simulink model "Gyro_Heading_Estimation"  (R2019a)
settings: Solver=ode3  StartTime=0.0  StopTime=inf  FixedStep=0.002  RelTol=1e-3  EnableMultiTasking=on
undefined symbols (not defined in the file): HIL, qc_get_step_size
libraries: quarc_library x12, simulink x8
settings Model: SimulationMode=external  ExtModeTrigDuration=10000  Creator=Derek  LastModifiedBy=Derek
settings SolverCC: PositivePriorityOrder=on
settings DataIOCC: ReturnWorkspaceOutputs=off
settings DebuggingCC: ArithmeticOperatorsInVariantConditions=warning
settings HardwareCC: ProdBitPerLong=64  ProdLargestAtomicInteger=LongLong  ProdLargestAtomicFloat=Double  ProdLongLongMode=on  ProdHWDeviceType=ARM Compatible->ARM 64-bit (LP64)
settings SFSimCC: SimUseLocalCustomCode=off
settings RTWCC: SystemTargetFile=quarc_linux_nvidia.tlc  TemplateMakefile=quarc_default_tmf  Description=QUARC Linux Nvidia Target (QCar) Using Toolchain  RTWUseLocalCustomCode=off  Toolchain=QUARC linux_nvidia | gmake (64-bit Windows)  BuildConfiguration=Faster Runs
settings CodeAppCC: StateflowObjectComments=on
settings STFCustomTargetCC: TargetLangStandard=C99 (ISO)  ConcurrentExecutionCompliant=on  UseToolchainInfoCompliant=on  SystemTargetFile=quarc_linux_nvidia.tlc
settings GRTTargetCC: ParMdlRefBuildCompliant=off  CompOptLevelCompliant=off  CombineOutputUpdateFcns=off  MatFileLogging=off  CPPClassGenCompliant=off  GRTInterface=on  ExtMode=on  ExtModeMexFile=quarc_comm  ExtModeMexArgs='-w -d /tmp -uri %u'
settings ConfigComp: CovMetricSettings=dswe

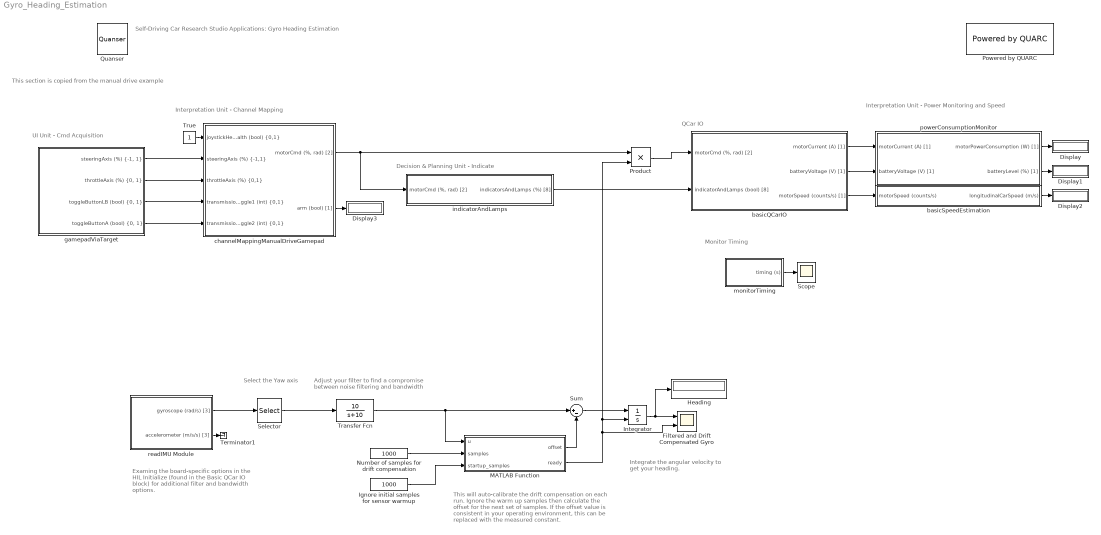
== system Gyro_Heading_Estimation ==
  note: Select the Yaw axis
  note: Decision & Planning Unit - Indicate
  note: Interpretation Unit - Power Monitoring and Speed
  note: QCar IO
  note: UI Unit - Cmd Acquisition
  note: Monitor Timing
  note: Interpretation Unit - Channel Mapping
  note: Self-Driving Car Research Studio
      | Applications: Gyro Heading Estimation
  note: This section is copied from the manual drive example
  note: Adjust your filter to find a compromise
      | between noise filtering and bandwidth
  note: This will auto-calibrate the drift compensation
      | on each run. Ignore the warm up samples
      | then calculate the offset for the next set of samples.
      | If the offset value is consistent in your operating
      | environment, this can be replaced with the measured
      | constant.
  note: Integrate the angular velocity to
      | get your heading.
  note: Examing the board-specific options
      | in the HIL Initialize (found in the Basic
      | QCar IO block) for additional filter
      | and bandwidth options.
  Display{,1..3} (4 alike) : Display
      Display settings: Decimation=0.5/qc_get_step_size
      Display1 settings: Decimation=0.5/qc_get_step_size
      Display2 settings: Decimation=0.5/qc_get_step_size
      Display3 settings: Decimation=0.1/qc_get_step_size
  Filtered and Drift Compensated Gyro : Scope  NumInputPorts=2
  Heading : Display
  Ignore initial samples for sensor warmup : Constant  Value=1000
  Integrator : Integrator  ExternalReset=rising
  MATLAB Function : MATLAB Function  TreatAsAtomicUnit=on
  Number of samples for drift compensation : Constant  Value=1000
  Powered by QUARC : quarc_library/Logos/Powered by QUARC
  Product : Product
  Quanser : quarc_library/Logos/Quanser
  Scope : Scope
  Selector : Selector  InputPortWidth=3  IndexOptions=Index vector (dialog)  Indices=[3]  OutputSizes=1
  Sum : Sum  Inputs=|+-
  Terminator1 : Terminator
  Transfer Fcn : TransferFcn  Numerator=[10]  Denominator=[1 10]
  True : Constant
  basicQCarIO : Subsystem
  basicSpeedEstimation : Subsystem
  channelMappingManualDriveGamepad : Subsystem
  gamepadViaTarget : Subsystem
  indicatorAndLamps : Subsystem
  "monitorTiming " : Subsystem
  powerConsumptionMonitor : Subsystem
  readIMU Module : Subsystem
  wires:
  readIMU Module/1(gyroscope (rad/s) [3]) -> Selector/1
  readIMU Module/2(accelerometer (m/s/s) [3]) -> Terminator1/1
  Selector/1 -> Transfer Fcn/1
  Transfer Fcn/1 -> Sum/1, MATLAB Function/1(u)
  Integrator/1 -> Heading/1, Filtered and Drift Compensated Gyro/1
  Sum/1 -> Integrator/1
  MATLAB Function/1(offset) -> Sum/2
  MATLAB Function/2(ready) -> Filtered and Drift Compensated Gyro/2, Product/2, Integrator/2
  Number of samples for drift compensation/1 -> MATLAB Function/2(samples)
  Ignore initial samples for sensor warmup/1 -> MATLAB Function/3(startup_samples)
  basicQCarIO/3(motorSpeed (counts/s) [1]) -> basicSpeedEstimation/1(motorSpeed (counts/s))
  gamepadViaTarget/4("toggleButtonA (bool) {0, 1}") -> channelMappingManualDriveGamepad/5("transmissionToggle2 (int) {0,1}")
  True/1 -> channelMappingManualDriveGamepad/1("joystickHealth (bool) {0,1}")
  gamepadViaTarget/1("steeringAxis (%) {-1, 1}") -> channelMappingManualDriveGamepad/2("steeringAxis (%) {-1,1}")
  basicQCarIO/1(motorCurrent (A) [1]) -> powerConsumptionMonitor/1(motorCurrent (A) [1])
  gamepadViaTarget/3("toggleButtonLB (bool) {0, 1}") -> channelMappingManualDriveGamepad/4("transmissionToggle1 (int) {0,1}")
  powerConsumptionMonitor/1(motorPowerConsumption (W) [1]) -> Display/1
  powerConsumptionMonitor/2(batteryLevel (%) [1]) -> Display1/1
  gamepadViaTarget/2("throttleAxis (%) {0, 1}") -> channelMappingManualDriveGamepad/3("throttleAxis (%) {0,1}")
  channelMappingManualDriveGamepad/1("motorCmd (%, rad) [2]") -> indicatorAndLamps/1("motorCmd (%, rad) [2]"), Product/1
  basicQCarIO/2(batteryVoltage (V) [1]) -> powerConsumptionMonitor/2(batteryVoltage (V) [1])
  basicSpeedEstimation/1(longitudinalCarSpeed (m/s)) -> Display2/1
  channelMappingManualDriveGamepad/2(arm (bool) [1]) -> Display3/1
  "monitorTiming "/1(timing (s)) -> Scope/1
  indicatorAndLamps/1(indicatorsAndLamps (%) [8]) -> basicQCarIO/2(indicatorAndLamps (bool) [8])
  Product/1 -> basicQCarIO/1("motorCmd (%, rad) [2]")

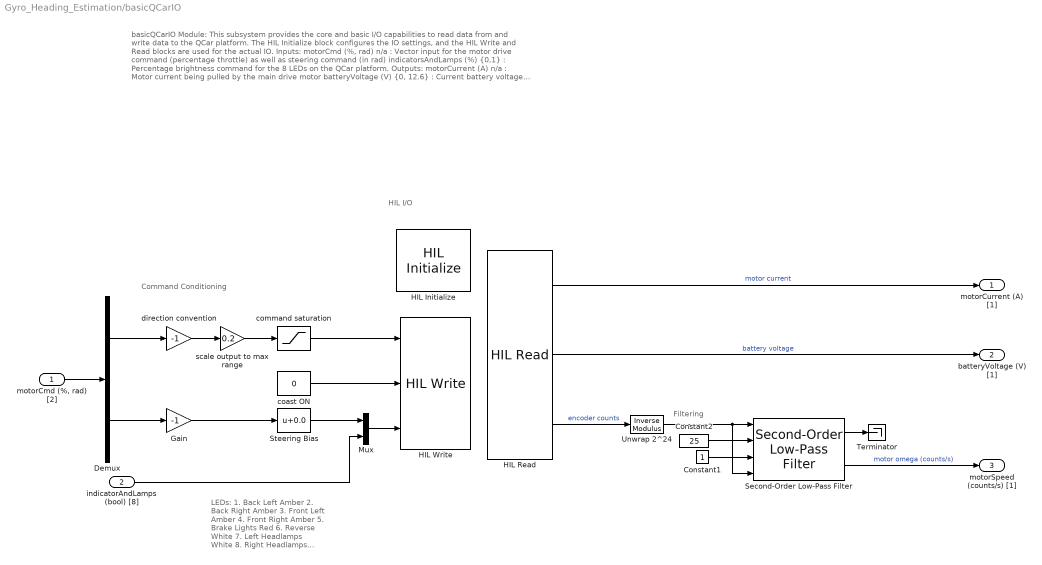
== system Gyro_Heading_Estimation/basicQCarIO ==
  note: Filtering
  note: basicQCarIO Module:
      |
      | This subsystem provides the core and basic I/O capabilities to read data from and write data to the QCar platform. The HIL Initialize block configures the IO settings, and the HIL Write and Read blocks are used for the actual IO.
      |
      | Inputs:
      | motorCmd (%, rad) n/a : Vector input for the motor drive command (percentage throttle) as well as steering command (in rad)
      | indicatorsAndLamps (%) {0,1} : Percentage brightness command for the 8 LEDs on the QCar platform.
      |
      | Outputs:
      | motorCurrent (A) n/a : Motor current being pulled by the main drive motor
      | batteryVoltage (V) {0, 12.6} : Current battery voltage reading
      | motorSpeed (counts/s) n/a : Drive motor speed measured using an encoder (do not confuse with wheel speed as this measurement is at the drive shaft)
  note: Command Conditioning
  note: HIL I/O
  note: LEDs:
      | 1. Back Left Amber
      | 2. Back Right Amber
      | 3. Front Left Amber
      | 4. Front Right Amber
      | 5. Brake Lights Red
      | 6. Reverse White
      | 7. Left Headlamps White
      | 8. Right Headlamps White
  "motorCmd (%, rad) [2]" : Inport
  indicatorAndLamps (bool) [8] : Inport  Port=2
  Constant1 : Constant
  Constant2 : Constant  Value=25
  Demux : Demux  Outputs=2
  Gain : Gain  Gain=-1
  HIL Initialize : quarc_library/Data Acquisition/Generic/Configuration/HIL Initialize  object_name=HIL-2  board_type=qcar  board_number=0  board_options=gyro_fs=250;gyro_rate=64;accel_fs=2;accel_rate=62.5;mag_rate=20;mag_xy=47;mag_z=83;enc1_dir=0;enc2_dir=0;enc3_dir=0;enc4_dir=0;pwm1_dshot=0;pwm2_dshot=0;pwm3_dshot=0;pwm4_dshot=0;pwm5_dshot=0;pwm6_dshot=0;pwm7_dshot=0;steer_bias=0.05;motor_limit=0.3;  exclusive=off  active=on  hardware_clocks=[]  clock_modes=[]  initial_clock_frequencies=[]  set_clock_params_at_start=off  set_clock_params_at_switch_in=off  set_clock_frequencies_at_start=off  set_clock_frequencies_at_switch_in=off  analog_input_channels=[0:6]  analog_input_configurations=[]  analog_input_maximums=[3.3]  analog_input_minimums=[0]  set_analog_input_params_at_start=off  set_analog_input_params_at_switch_in=off  analog_output_channels=[]  analog_output_maximums=[]  analog_output_minimums=[]  initial_analog_outputs=[]  final_analog_outputs=[]  watchdog_analog_outputs=[]  set_analog_output_params_at_start=off  set_analog_output_params_at_switch_in=off  set_analog_outputs_at_start=off  set_analog_outputs_at_switch_in=off  set_analog_outputs_at_terminate=off  set_analog_outputs_at_switch_out=off  set_analog_outputs_on_watchdog=off  digital_input_channels=[24:43]  digital_output_channels=[40]  digital_output_configuration=[]  initial_digital_outputs=[0]  final_digital_outputs=[1]  watchdog_digital_outputs=[]  set_digital_output_params_at_start=off  set_digital_output_params_at_switch_in=off  set_digital_outputs_at_start=on  set_digital_outputs_at_switch_in=off  set_digital_outputs_at_terminate=on  set_digital_outputs_at_switch_out=off  set_digital_outputs_on_watchdog=off  encoder_channels=[0:4]  quadrature=[4 4]  encoder_filter_frequency=100e6/1  initial_encoder_counts=[0]  set_encoder_params_at_start=on  set_encoder_params_at_switch_in=off  set_encoder_counts_at_start=on  set_encoder_counts_at_switch_in=off  pwm_channels=[0:7]  pwm_modes=[0 0]  pwm_frequency=150e6/4096  pwm_configuration=[0]  pwm_alignment=[0]  pwm_polarity=[1]  pwm_leading_deadband=[]  pwm_trailing_deadband=[]  initial_pwm_outputs=[0]  final_pwm_outputs=[0]  watchdog_pwm_outputs=[0]  set_pwm_params_at_start=on  set_pwm_params_at_switch_in=off  set_pwm_outputs_at_start=on  set_pwm_outputs_at_switch_in=off  set_pwm_outputs_at_terminate=on  set_pwm_outputs_at_switch_out=off  set_pwm_outputs_on_watchdog=off  other_output_channels=[1000, 11000:11011]  initial_other_outputs=[0]  final_other_outputs=[0]  watchdog_other_outputs=[]  set_other_outputs_at_start=on  set_other_outputs_at_switch_in=off  set_other_outputs_at_terminate=on  set_other_outputs_at_switch_out=off  set_other_outputs_on_watchdog=off
  HIL Read : quarc_library/Data Acquisition/Generic/Immediate I//O/HIL Read  object_name=HIL-2  analog_channels=[5:6]  encoder_channels=[0]  digital_channels=[]  other_channels=[]  sample_time=qc_get_step_size  active=on  vector_output=off  data_type_mode=Inherit via back propagation  encoder_data_type=double  digital_data_type=boolean
  HIL Write : quarc_library/Data Acquisition/Generic/Immediate I//O/HIL Write  object_name=HIL-2  analog_channels=[]  pwm_channels=[0]  digital_channels=[40]  other_channels=[1000 11008:11011 11000:11003]  sample_time=-1  active=off  vector_input=on
  Mux : Mux  Inputs=2
  Second-Order Low-Pass Filter : quarc_library/Continuous/Second-Order Low-Pass Filter  params_source=External (input ports)  input_width=1  input_zeta=1  input_init=0
  Steering Bias : Bias  Bias=0.0
  Terminator : Terminator
  Unwrap 2^24 : quarc_library/Discontinuities/Inverse Modulus  modulus=16777215  output_derivative=off  output_revolutions=off  max_x=Inf  min_x=-Inf
  coast ON : Constant  Value=0
  command saturation : Saturate  UpperLimit=0.20  LowerLimit=-0.20
  direction convention : Gain  Gain=-1
  scale output to max range : Gain  Gain=0.2
  motorCurrent (A) [1] : Outport
  batteryVoltage (V) [1] : Outport  Port=2
  motorSpeed (counts/s) [1] : Outport  Port=3
  wires:
  Constant2/1 -> Second-Order Low-Pass Filter/2
  Unwrap 2^24/1 -> Second-Order Low-Pass Filter/1, Second-Order Low-Pass Filter/4
  Demux/2 -> Gain/1
  direction convention/1 -> scale output to max range/1
  "motorCmd (%, rad) [2]"/1 -> Demux/1
  command saturation/1 -> HIL Write/1
  coast ON/1 -> HIL Write/2
  Second-Order Low-Pass Filter/1 -> Terminator/1
  indicatorAndLamps (bool) [8]/1 -> Mux/2
  Steering Bias/1 -> Mux/1
  Mux/1 -> HIL Write/3
  Second-Order Low-Pass Filter/2 -> motorSpeed (counts/s) [1]/1  "motor omega (counts/s)"
  Constant1/1 -> Second-Order Low-Pass Filter/3
  Demux/1 -> direction convention/1
  HIL Read/3 -> Unwrap 2^24/1  "encoder counts"
  Gain/1 -> Steering Bias/1
  HIL Read/1 -> motorCurrent (A) [1]/1  "motor current"
  HIL Read/2 -> batteryVoltage (V) [1]/1  "battery voltage"
  scale output to max range/1 -> command saturation/1

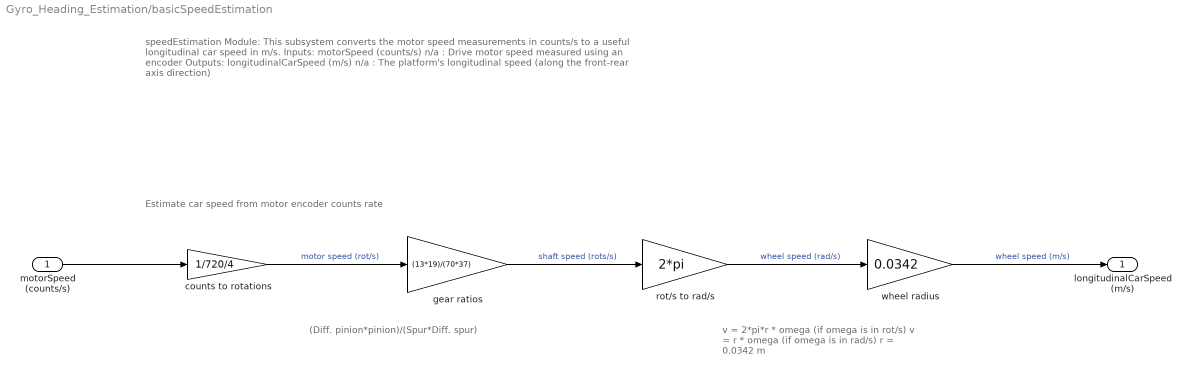
== system Gyro_Heading_Estimation/basicSpeedEstimation ==
  note: speedEstimation Module:
      |
      | This subsystem converts the motor speed measurements in counts/s to a useful longitudinal car speed in m/s.
      |
      | Inputs:
      | motorSpeed (counts/s) n/a : Drive motor speed measured using an encoder
      |
      | Outputs:
      | longitudinalCarSpeed (m/s) n/a : The platform's longitudinal speed (along the front-rear axis direction)
  note: (Diff. pinion*pinion)/(Spur*Diff. spur)
  note: v = 2*pi*r * omega (if omega is in rot/s)
      | v = r * omega (if omega is in rad/s)
      | r = 0.0342 m
  note: Estimate car speed from motor encoder counts rate
  motorSpeed (counts/s) : Inport
  counts to rotations : Gain  Gain=1/720/4
  gear ratios : Gain  Gain=(13*19)/(70*37)
  rot/s to rad/s : Gain  Gain=2*pi
  wheel radius : Gain  Gain=0.0342
  longitudinalCarSpeed (m/s) : Outport
  wires:
  gear ratios/1 -> rot/s to rad/s/1  "shaft speed (rots/s)"
  wheel radius/1 -> longitudinalCarSpeed (m/s)/1  "wheel speed (m/s)"
  counts to rotations/1 -> gear ratios/1  "motor speed (rot/s)"
  rot/s to rad/s/1 -> wheel radius/1  "wheel speed (rad/s)"
  motorSpeed (counts/s)/1 -> counts to rotations/1

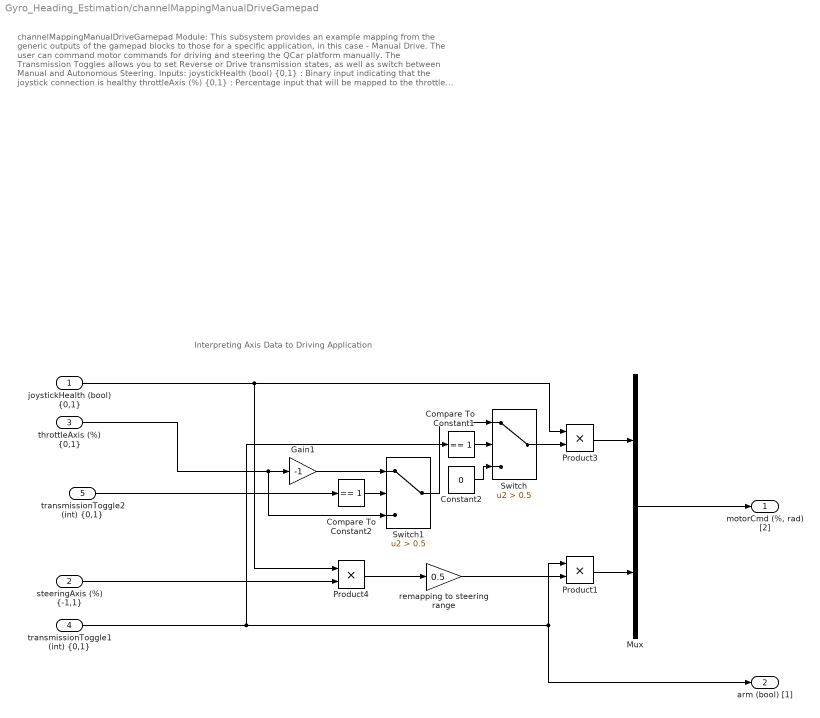
== system Gyro_Heading_Estimation/channelMappingManualDriveGamepad ==
  note: channelMappingManualDriveGamepad Module:
      |
      | This subsystem provides an example mapping from the generic outputs of the gamepad blocks to those for a specific application, in this case - Manual Drive. The user can command motor commands for driving and steering the QCar platform manually. The Transmission Toggles allows you to set Reverse or Drive transmission states, as well as switch between Manual and Autonomous Steering.
      |
      | Inputs:
      | joystickHealth (bool) {0,1} : Binary input indicating that the joystick connection is healthy
      | throttleAxis (%) {0,1} : Percentage input that will be mapped to the throttle command
      | steeringAxis (%) {-1,1} : Signed percentage input that will be mapped to steering
      | transmissionToggle1 (int) {0,1} : 2-state input that will decide the Park/Engage State
      | transmissionToggle2 (int) {0, 1} : 2-state input that will decide the Reverse/Drive State
      |
      | Outputs:
      | motorCmd (%, rad) n/a : Vector output for the motor drive command (percentage throttle) as well as steering command (in rad)
      | arm (bool) {0,1} : Binary output indicating status (armed or disarmed)
      |
      | Usage:
      | 1. When the Transmission Toggle 1 input
      | a. reads 1, the Arm output will be high (1), which is the Armed state.
      | b. reads 0, the Arm output will be low (0), which is the Disarmed state.
      | 2. In addition, the Transmission Toggle 2 input
      | a. reading 0 is the Drive state, and the Motor Cmd for the throttle will range from 0 to 100%, spinning the wheels forwards.
      | b. reading 1 is the Reverse state, and the Motor Cmd for the throttle will range from 0 to -100%, spinning the wheels backwards.
  note: Interpreting Axis Data to Driving Application
  "joystickHealth (bool) {0,1}" : Inport
  "steeringAxis (%) {-1,1}" : Inport  Port=2
  "throttleAxis (%) {0,1}" : Inport  Port=3
  "transmissionToggle1 (int) {0,1}" : Inport  Port=4
  "transmissionToggle2 (int) {0,1}" : Inport  Port=5
  " remapping to steering range " : Gain  Gain=0.5
  Compare To Constant1 : simulink/Logic and Bit Operations/Compare To Constant  relop===  const=1  OutDataTypeStr=boolean
  Compare To Constant2 : simulink/Logic and Bit Operations/Compare To Constant  relop===  const=1  OutDataTypeStr=boolean
  Constant2 : Constant  Value=0
  Gain1 : Gain  Gain=-1
  Mux : Mux  Inputs=2
  Product1 : Product
  Product3 : Product
  Product4 : Product
  Switch : Switch  Criteria=u2 > Threshold  Threshold=0.5
  Switch1 : Switch  Criteria=u2 > Threshold  Threshold=0.5
  "motorCmd (%, rad) [2]" : Outport
  arm (bool) [1] : Outport  Port=2
  wires:
  Switch/1 -> Product3/2
  Product1/1 -> Mux/2
  Compare To Constant1/1 -> Switch/2
  "steeringAxis (%) {-1,1}"/1 -> Product4/2
  "joystickHealth (bool) {0,1}"/1 -> Product4/1, Product3/1
  "transmissionToggle1 (int) {0,1}"/1 -> Compare To Constant1/1, Product1/1, arm (bool) [1]/1
  Product3/1 -> Mux/1
  " remapping to steering range "/1 -> Product1/2
  Product4/1 -> " remapping to steering range "/1
  "throttleAxis (%) {0,1}"/1 -> Switch1/3, Gain1/1
  Mux/1 -> "motorCmd (%, rad) [2]"/1
  Compare To Constant2/1 -> Switch1/2
  Switch1/1 -> Switch/1
  Constant2/1 -> Switch/3
  "transmissionToggle2 (int) {0,1}"/1 -> Compare To Constant2/1
  Gain1/1 -> Switch1/1

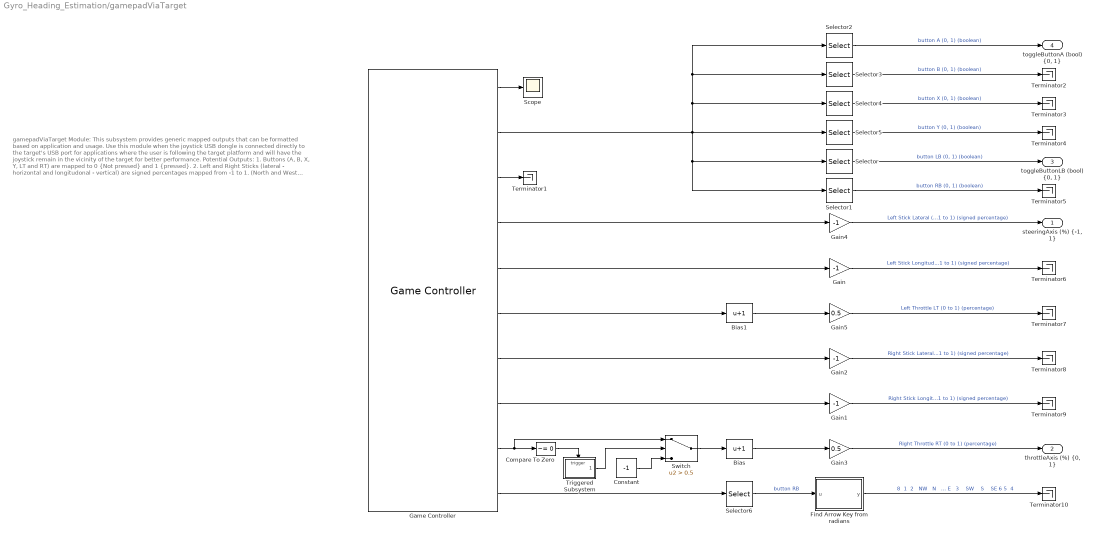
== system Gyro_Heading_Estimation/gamepadViaTarget ==
  note: gamepadViaTarget Module:
      |
      | This subsystem provides generic mapped outputs that can be formatted based on application and usage. Use this module when the joystick USB dongle is connected directly to the target's USB port for applications where the user is following the target platform and will have the joystick remain in the vicinity of the target for better performance.
      |
      | Potential Outputs:
      |
      | 1. Buttons (A, B, X, Y, LT and RT) are mapped to 0 {Not pressed} and 1 {pressed}.
      |
      | 2. Left and Right Sticks (lateral - horizontal and longitudonal - vertical) are signed percentages mapped from -1 to 1. (North and West directions are positive)
      |
      | 3. Throttle (RT and LT) are mapped from 0 to 1.
      |
      | 4. Arrow keys are mapped to constants 1 to 8 starting from North and incrementing clockwise up to North West. A value of 0 implies no keys are pressed.
      |
      | 5. The NEW signal triggers a high (1) pulse whenever a value on any of the gamepad's keys changes.
      |
      | NOTE: The Gamepad F710 dongle MUST be plugged into the target's USB port to use this module.
  Bias : Bias  Bias=1
  Bias1 : Bias  Bias=1
  Compare To Zero : simulink/Logic and Bit Operations/Compare To Zero  relop=~=  OutDataTypeStr=boolean
  Constant : Constant  Value=-1
  Find Arrow Key from radians : MATLAB Function  TreatAsAtomicUnit=on
  Gain{,1..2,4} (4 alike) : Gain  Gain=-1
  Gain3 : Gain  Gain=0.5
  Gain5 : Gain  Gain=0.5
  Game Controller : quarc_library/Devices/Peripherals/Target/Game Controller  controller=1  buffer_size=12  deadzone=[]  saturation=[]  sample_time=qc_get_step_size  auto_center=off  enabled=on
      settings: SourceProductName=QUARC Targets
  Scope : Scope
  Selector : Selector  InputPortWidth=32  IndexOptions=Index vector (dialog)  Indices=[5]  OutputSizes=1
  Selector1 : Selector  InputPortWidth=32  IndexOptions=Index vector (dialog)  Indices=[6]  OutputSizes=1
  Selector2 : Selector  InputPortWidth=32  IndexOptions=Index vector (dialog)  Indices=[1]  OutputSizes=1
  Selector3 : Selector  InputPortWidth=32  IndexOptions=Index vector (dialog)  Indices=[2]  OutputSizes=1
  Selector4 : Selector  InputPortWidth=32  IndexOptions=Index vector (dialog)  Indices=[3]  OutputSizes=1
  Selector5 : Selector  InputPortWidth=32  IndexOptions=Index vector (dialog)  Indices=[4]  OutputSizes=1
  Selector6 : Selector  InputPortWidth=4  IndexOptions=Index vector (dialog)  Indices=[1]  OutputSizes=1
  Switch : Switch  Criteria=u2 > Threshold  Threshold=0.5
  Terminator{1..10} (10 alike) : Terminator
  Triggered Subsystem : Subsystem  TreatAsAtomicUnit=on
  "steeringAxis (%) {-1, 1}" : Outport
  "throttleAxis (%) {0, 1}" : Outport  Port=2
  "toggleButtonLB (bool) {0, 1}" : Outport  Port=3
  "toggleButtonA (bool) {0, 1}" : Outport  Port=4
  wires:
  Gain5/1 -> Terminator7/1  "Left Throttle LT (0 to 1) (percentage)"
  Bias1/1 -> Gain5/1
  Game Controller/6 -> Bias1/1
  Game Controller/10 -> Selector6/1
  Selector5/1 -> Terminator4/1  "button Y (0, 1) (boolean)"
  Selector4/1 -> Terminator3/1  "button X (0, 1) (boolean)"
  Selector3/1 -> Terminator2/1  "button B (0, 1) (boolean)"
  Game Controller/1 -> Scope/1
  Game Controller/5 -> Gain/1
  Game Controller/4 -> Gain4/1
  Game Controller/8 -> Gain1/1
  Game Controller/7 -> Gain2/1
  Game Controller/2 -> Selector1/1, Selector/1, Selector5/1, Selector2/1, Selector3/1, Selector4/1
  Bias/1 -> Gain3/1
  Gain2/1 -> Terminator8/1  "Right Stick Lateral (-1 to 1) (signed percentage)"
  Gain1/1 -> Terminator9/1  "Right Stick Longitudonal (-1 to 1) (signed percentage)"
  Gain/1 -> Terminator6/1  "Left Stick Longitudonal (-1 to 1) (signed percentage)"
  Selector1/1 -> Terminator5/1  "button RB (0, 1) (boolean)"
  Selector/1 -> "toggleButtonLB (bool) {0, 1}"/1  "button LB (0, 1) (boolean)"
  Gain3/1 -> "throttleAxis (%) {0, 1}"/1  "Right Throttle RT (0 to 1) (percentage)"
  Selector2/1 -> "toggleButtonA (bool) {0, 1}"/1  "button A (0, 1) (boolean)"
  Gain4/1 -> "steeringAxis (%) {-1, 1}"/1  "Left Stick Lateral (-1 to 1) (signed percentage)"
  Selector6/1 -> Find Arrow Key from radians/1(u)  "button RB"
  Find Arrow Key from radians/1(y) -> Terminator10/1  "8 \t\t\t1\t\t\t 2   NW\t  N\t\t  NE \t\t 7     W\t\t0\t\t  E   3     SW\t   S\t\t   SE 6\t\t\t5\t\t\t 4"
  Game Controller/3 -> Terminator1/1
  Switch/1 -> Bias/1
  Game Controller/9 -> Switch/1, Compare To Zero/1
  Triggered Subsystem/1(Enabled) -> Switch/2
  Constant/1 -> Switch/3
  Compare To Zero/1 -> Triggered Subsystem/Trigger

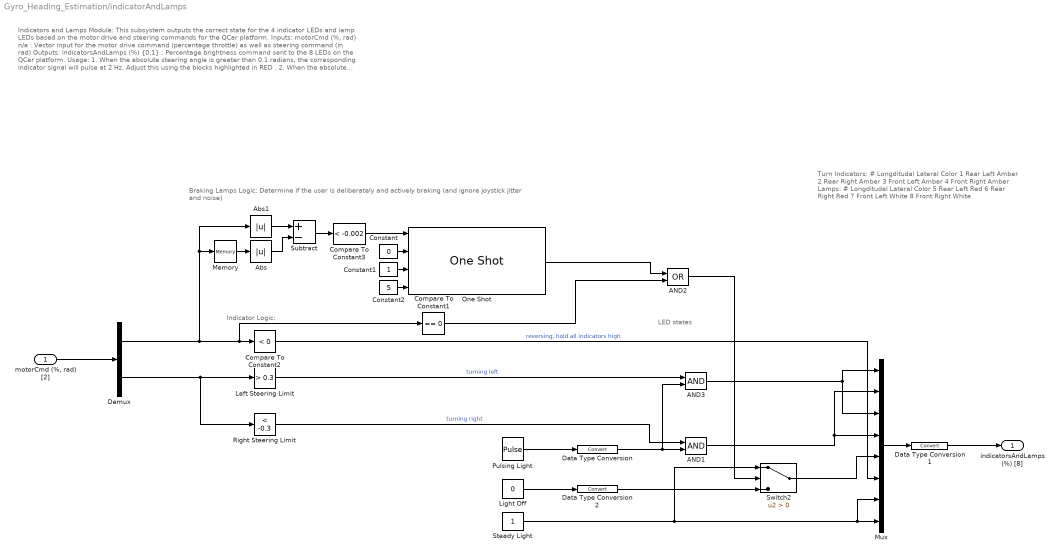
== system Gyro_Heading_Estimation/indicatorAndLamps ==
  note: Indicators and Lamps Module:
      |
      | This subsystem outputs the correct state for the 4 indicator LEDs and lamp LEDs based on the motor drive and steering commands for the QCar platform.
      |
      | Inputs:
      | motorCmd (%, rad) n/a : Vector input for the motor drive command (percentage throttle) as well as steering command (in rad)
      |
      | Outputs:
      | indicatorsAndLamps (%) {0,1} : Percentage brightness command sent to the 8 LEDs on the QCar platform.
      |
      | Usage:
      | 1. When the absolute steering angle is greater than 0.1 radians, the corresponding indicator signal will pulse at 2 Hz. Adjust this using the blocks highlighted in RED .
      | 2. When the absolute motor drive command approaches 0, the brake lamps will receive 100% brightness command, and 0% brightness otherwise. Adjust this using the blocks highlighted in GREEN .
  note: Braking Lamps Logic:
      | Determine if the user is deliberately and actively braking (and ignore joystick jitter and noise)
  note: LED states
  note: Turn Indicators:
      | # Longditudal Lateral Color
      | 1 Rear Left Amber
      | 2 Rear Right Amber
      | 3 Front Left Amber
      | 4 Front Right Amber
      |
      | Lamps:
      | # Longditudal Lateral Color
      | 5 Rear Left Red
      | 6 Rear Right Red
      | 7 Front Left White
      | 8 Front Right White
  note: Indicator Logic:
  "motorCmd (%, rad) [2]" : Inport
  AND1 : Logic  IconShape=distinctive  AllPortsSameDT=off  OutDataTypeStr=boolean
  AND2 : Logic  Operator=OR  IconShape=distinctive  AllPortsSameDT=off  OutDataTypeStr=boolean
  AND3 : Logic  IconShape=distinctive  AllPortsSameDT=off  OutDataTypeStr=boolean
  Abs : Abs
  Abs1 : Abs
  Compare To Constant1 : simulink/Logic and Bit Operations/Compare To Constant  relop===  const=0  OutDataTypeStr=uint8
  Compare To Constant2 : simulink/Logic and Bit Operations/Compare To Constant  relop=<  const=0  OutDataTypeStr=boolean
  Compare To Constant3 : simulink/Logic and Bit Operations/Compare To Constant  relop=<  const=-0.002  OutDataTypeStr=boolean
  Constant : Constant  Value=0
  Constant1 : Constant
  Constant2 : Constant  Value=5
  Data Type Conversion : DataTypeConversion
  Data Type Conversion1 : DataTypeConversion
  Data Type Conversion2 : DataTypeConversion
  Demux : Demux  Outputs=2
  Left Steering Limit : simulink/Logic and Bit Operations/Compare To Constant  relop=>  const=0.3  OutDataTypeStr=boolean
  Light Off : Constant  Value=0  OutDataTypeStr=boolean
  Memory : Memory
  Mux : Mux  Inputs=8
  One Shot : quarc_library/Discontinuities/One Shot  trigger_type=Falling edge  redun_pulse=Ignore extraneous pulse  width_source=External input port  pulse_width=100
      settings: SourceProductName=QUARC Targets
  Pulsing Light : DiscretePulseGenerator  Period=0.5/qc_get_step_size  PulseWidth=0.5/2/qc_get_step_size  SampleTime=qc_get_step_size
  Right Steering Limit : simulink/Logic and Bit Operations/Compare To Constant  relop=<  const=-0.3  OutDataTypeStr=boolean
  Steady Light : Constant  OutDataTypeStr=boolean
  Subtract : Sum  Inputs=+-
  Switch2 : Switch  Criteria=u2 > Threshold
  indicatorsAndLamps (%) [8] : Outport
  wires:
  Data Type Conversion2/1 -> Switch2/3
  Demux/2 -> Right Steering Limit/1, Left Steering Limit/1
  Light Off/1 -> Data Type Conversion2/1
  One Shot/1 -> AND2/1
  Steady Light/1 -> Mux/7, Mux/8, Switch2/1
  Compare To Constant3/1 -> One Shot/1
  Constant2/1 -> One Shot/4
  Right Steering Limit/1 -> AND1/1  "turning right"
  Mux/1 -> Data Type Conversion1/1
  Constant/1 -> One Shot/2
  Pulsing Light/1 -> Data Type Conversion/1
  Abs/1 -> Subtract/2
  Memory/1 -> Abs/1
  Abs1/1 -> Subtract/1
  Data Type Conversion/1 -> AND3/2, AND1/2
  Data Type Conversion1/1 -> indicatorsAndLamps (%) [8]/1
  Left Steering Limit/1 -> AND3/1  "turning left"
  Switch2/1 -> Mux/5
  Constant1/1 -> One Shot/3
  Demux/1 -> Compare To Constant1/1, Compare To Constant2/1, Memory/1, Abs1/1
  AND3/1 -> Mux/1, Mux/3
  "motorCmd (%, rad) [2]"/1 -> Demux/1
  Subtract/1 -> Compare To Constant3/1
  AND1/1 -> Mux/2, Mux/4
  Compare To Constant2/1 -> Mux/6  "reversing, hold all indicators high"
  Compare To Constant1/1 -> AND2/2
  AND2/1 -> Switch2/2

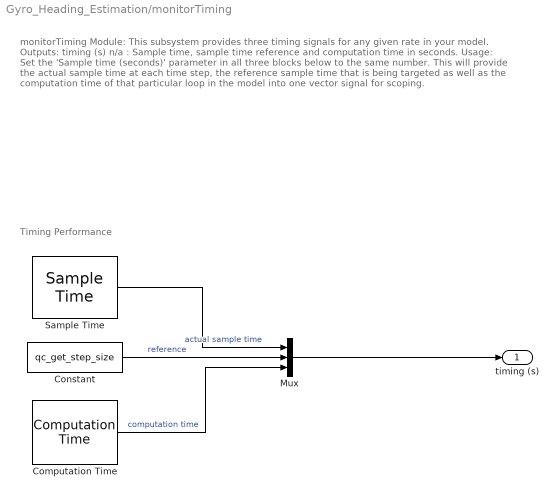
== system Gyro_Heading_Estimation/monitorTiming  ==
  note: Timing Performance
  note: monitorTiming Module:
      |
      | This subsystem provides three timing signals for any given rate in your model.
      |
      | Outputs:
      | timing (s) n/a : Sample time, sample time reference and computation time in seconds.
      |
      | Usage:
      | Set the 'Sample time (seconds)' parameter in all three blocks below to the same number. This will provide the actual sample time at each time step, the reference sample time that is being targeted as well as the computation time of that particular loop in the model into one vector signal for scoping.
  Computation Time : quarc_library/Sources/Time/Computation Time  sample_time=qc_get_step_size  use_model=on  use_cpu_time=off
  Constant : Constant  Value=qc_get_step_size
  Mux : Mux  Inputs=3
  Sample Time : quarc_library/Sources/Time/Sample Time  Priority=-99  sample_time=qc_get_step_size
  timing (s) : Outport
  wires:
  Mux/1 -> timing (s)/1
  Computation Time/1 -> Mux/3  "computation time"
  Sample Time/1 -> Mux/1  "actual sample time"
  Constant/1 -> Mux/2  "reference"

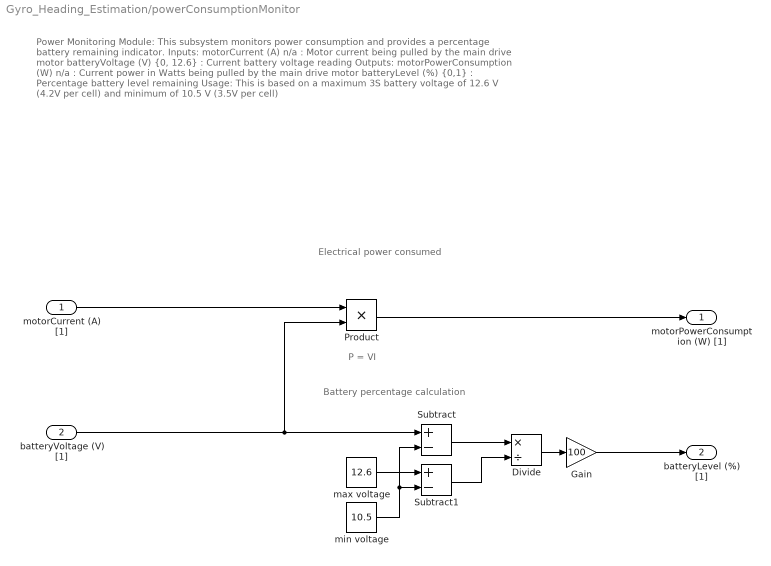
== system Gyro_Heading_Estimation/powerConsumptionMonitor ==
  note: Battery percentage calculation
  note: P = VI
  note: Electrical
      | power
      | consumed
  note: Power Monitoring Module:
      |
      | This subsystem monitors power consumption and provides a percentage battery remaining indicator.
      |
      | Inputs:
      | motorCurrent (A) n/a : Motor current being pulled by the main drive motor
      | batteryVoltage (V) {0, 12.6} : Current battery voltage reading
      |
      | Outputs:
      | motorPowerConsumption (W) n/a : Current power in Watts being pulled by the main drive motor
      | batteryLevel (%) {0,1} : Percentage battery level remaining
      |
      | Usage:
      | This is based on a maximum 3S battery voltage of 12.6 V (4.2V per cell) and minimum of 10.5 V (3.5V per cell)
  motorCurrent (A) [1] : Inport
  batteryVoltage (V) [1] : Inport  Port=2
  Divide : Product  Inputs=*/
  Gain : Gain  Gain=100
  Product : Product
  Subtract : Sum  Inputs=+-
  Subtract1 : Sum  Inputs=+-
  max voltage : Constant  Value=12.6
  min voltage : Constant  Value=10.5
  motorPowerConsumption (W) [1] : Outport
  batteryLevel (%) [1] : Outport  Port=2
  wires:
  Divide/1 -> Gain/1
  Subtract1/1 -> Divide/2
  Gain/1 -> batteryLevel (%) [1]/1
  Product/1 -> motorPowerConsumption (W) [1]/1
  min voltage/1 -> Subtract/2, Subtract1/2
  motorCurrent (A) [1]/1 -> Product/1
  max voltage/1 -> Subtract1/1
  Subtract/1 -> Divide/1
  batteryVoltage (V) [1]/1 -> Subtract/1, Product/2

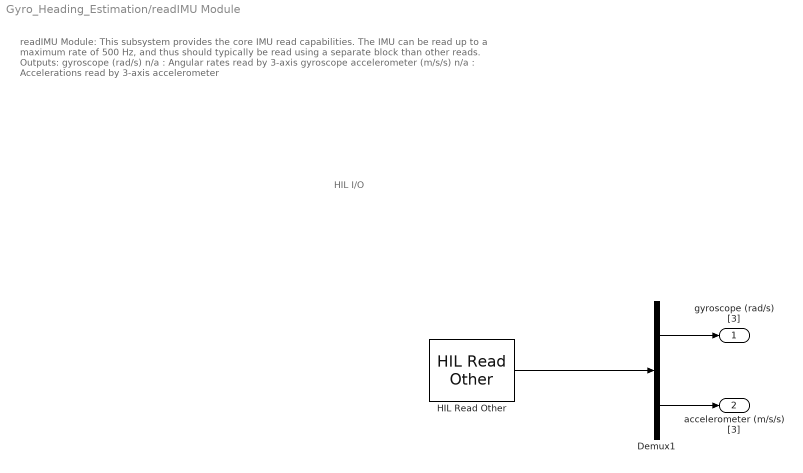
== system Gyro_Heading_Estimation/readIMU Module ==
  note: readIMU Module:
      |
      | This subsystem provides the core IMU read capabilities. The IMU can be read up to a maximum rate of 500 Hz, and thus should typically be read using a separate block than other reads.
      |
      | Outputs:
      | gyroscope (rad/s) n/a : Angular rates read by 3-axis gyroscope
      | accelerometer (m/s/s) n/a : Accelerations read by 3-axis accelerometer
  note: HIL I/O
  Demux1 : Demux  Outputs=[3 3]
  HIL Read Other : quarc_library/Data Acquisition/Generic/Immediate I//O/HIL Read Other  object_name=HIL-2  channels=[3000:3002 4000:4002]  sample_time=qc_get_step_size  active=on  vector_output=on
      settings: AttributesFormatString=(%<object_name>)  SourceProductName=QUARC Targets
  gyroscope (rad/s) [3] : Outport
  accelerometer (m/s/s) [3] : Outport  Port=2
  wires:
  HIL Read Other/1 -> Demux1/1
  Demux1/1 -> gyroscope (rad/s) [3]/1
  Demux1/2 -> accelerometer (m/s/s) [3]/1

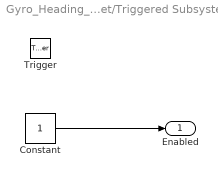
== system Gyro_Heading_Estimation/gamepadViaTarget/Triggered Subsystem ==
  Trigger : TriggerPort  VariantControl=Variant
  Constant : Constant
  Enabled : Outport  InitialOutput=[0]  VectorParamsAs1DForOutWhenUnconnected=on
  wires:
  Constant/1 -> Enabled/1

== matlab function Gyro_Heading_Estimation/gamepadViaTarget/Find Arrow Key from radians ==
  data: u input; y output
function y = fcn(u)

% the input signal gives the positon of the arrow keys pressed on the gamepad
% in radians circulating clockwise. Thus, up arrow alone is 0, right would be
% pi/2, and both up and right arrows pressed simultaneously is pi/4.
% 
% Given the input signal, convert to degrees for ease, then subtract the 
% vector 45*[0 1 2 3 4 5 6 7] to find smallest error corresponding to arrow
% pressed. 
if u == -1
    y = 0;
else
    [~, y] = min(abs((u*360/(2*pi)) - 45*[0 1 2 3 4 5 6 7]));
end

== matlab function Gyro_Heading_Estimation/MATLAB Function ==
  settings: updateMethod=DISCRETE
  data: u input; offset output; samples input; ready output; startup_samples input
function [offset, ready] = fcn(u, samples, startup_samples)

persistent sample_sum;
persistent remaining_samples;
persistent last_offset;
persistent last_ready;
persistent remaining_startup_samples;

if isempty(sample_sum)
    sample_sum = 0;
    remaining_samples = samples;
    remaining_startup_samples = startup_samples;
    last_offset = 0;
    last_ready = 0;
end

if (remaining_startup_samples > 0)
    remaining_startup_samples = remaining_startup_samples - 1;
else
    if (remaining_samples > 0) && (samples > 0)
        sample_sum = sample_sum + u;
        remaining_samples = remaining_samples - 1;

        if remaining_samples == 0
            last_offset = sample_sum/samples;
            last_ready = 1;
        end
    end
end

offset = last_offset;
ready = last_ready;
